simulink model "Lab1_419_simul"  (R2023b)
settings: Solver=VariableStepAuto  StartTime=0.0  StopTime=120  RelTol=1e-9
settings Model: Creator=Aiden  LastModifiedBy=Aiden

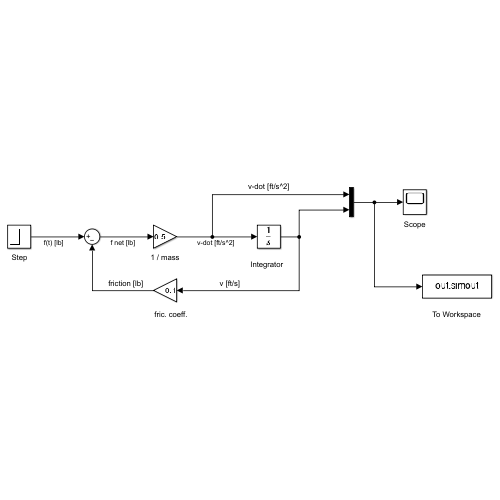
[thumbnail: Simulink's stored preview of the top-level diagram]
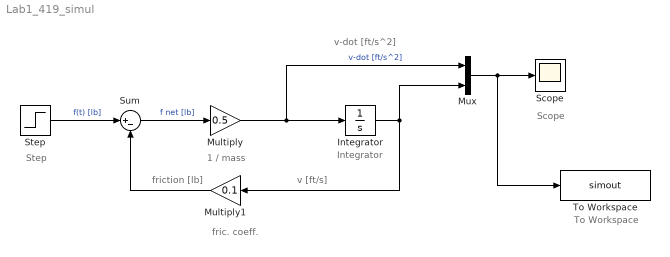
== system Lab1_419_simul ==
  note: 1 / mass
  note: v-dot [ft/s^2]
  note: fric. coeff.
  note: v [ft/s]
  note: friction [lb]
  note: To Workspace
  note: Integrator
  note: Scope
  note: Step
  Integrator : Integrator
  Multiply : Gain  Gain=0.5
  Multiply1 : Gain  Gain=0.1
  Mux : Mux  Inputs=2
  Scope : Scope
  Step : Step  SampleTime=0
  Sum : Sum  Inputs=|+-
  To Workspace : ToWorkspace  VariableName=simout  SampleTime=-1
  wires:
  Integrator/1 -> Multiply1/1, Mux/2
  Multiply/1 -> Mux/1, Integrator/1  "v-dot [ft/s^2]"
  Sum/1 -> Multiply/1  "f net [lb]"
  Multiply1/1 -> Sum/2
  Step/1 -> Sum/1  "f(t) [lb]"
  Mux/1 -> To Workspace/1, Scope/1
